simulink model "sm_motor_grader_Blade"  (R2025b)
settings: Solver=ode23t  StartTime=0.0  StopTime=stopTime  RelTol=1e-3  AbsTol=1e-3  EnableMultiTasking=on
undefined symbols (not defined in the file): activeTestCmds, motGradParams, X, Y, Z
libraries: sm_motor_grader_lib x4, sm_lib x4, nesl_utility x1, simulink x1
Description:
  | Copyright 2025 The MathWorks, Inc.
settings Model: Creator=smiller  LastModifiedBy=smiller
settings SolverCC: AutoScaleAbsTol=off  AlgebraicLoopSolver=TrustRegion  MaxZcPerStep=1.0
settings DataIOCC: LimitDataPoints=on  MaxDataPoints=10000  ReturnWorkspaceOutputs=off  SignalLoggingName=logsout_sm_motor_grader_Blade
settings OptimizationCC: ReuseModelBlockBuffer=off  LifeSpan=inf
settings DebuggingCC: UnconnectedInputMsg=warning  UnconnectedOutputMsg=warning  UnconnectedLineMsg=warning  AllowSymbolicDim=off  SubsystemReferenceDiagnosticForUnitTest=warning  SFUnexpectedBacktrackingDiag=warning  SFNoUnconditionalDefaultTransitionDiag=warning  SFExecutionAtInitializationDiag=none  ArithmeticOperatorsInVariantConditions=warning
settings ModelReferenceCC: EnableRefExpFcnMdlSchedulingChecks=on
settings SFSimCC: SimUseLocalCustomCode=off  CustomCodeUndefinedFunction=UseInterfaceOnly
settings RTWCC: RTWUseLocalCustomCode=off  GPUComputeCapability=3.5  DLArmComputeVersion=19.05
settings CodeAppCC: StateflowObjectComments=on
settings GRTTargetCC: TargetLangStandard=C89/C90 (ANSI)
settings ConfigComp: CovMetricSettings=dw  CovSaveCumulativeToWorkspaceVar=on  CovSaveSingleToWorkspaceVar=on  CovExternalEMLEnable=off  CovSFcnEnable=off
settings SimscapeCC: SimscapeLogType=all  SimscapeLogSimulationStatistics=on  SimscapeLogName=simlog_sm_motor_grader_Blade  SimscapeLogLimitData=off  SimscapeLogDataHistory=10000.0
settings DiagnosticsConfigSet: SimMechanicsConflictingReferenceFrames=none
settings ExplorerConfigSet: InternalSimMechanicsExplorerSettings="<ExplorerConfiguration><canonicalview>default</canonicalview><AnimationSetting><BasePlaybackSpeed>1.0</BasePlaybackSpeed><PlaybackSpeedFactor>1.0</PlaybackSpeedFactor></AnimationSetting><TilePanel><TileInfo><Tiles Columns=\"1\" Count=\"1\" Rows=\"1\"><Column Weight=\"1\"/><Row Weight=\"1\"/><Tile Height=\"1\" Width=\"1\" X=\"0\" Y=\"0\"/></Tiles></TileInfo><SceneInfo><SceneViewer><BGColor><R>1</R><G>1</G><B>1</B></BGColor><Camera><DoPerspective>off</DoPerspective><Position><X>-3.46230362549575776</X><Y>-2.62208562860429995</Y><Z>1.68751467196826876</Z></Position><Center><X>-0.265224461381971088</X><Y>0.208729678692644943</Y><Z>0.662364084836305378</Z></Center><Up><X>0.210150762827159998</X><Y>0.114284437926875038</Y><Z>0.970966386715266694</Z></Up><ViewLimDist>1</ViewLimDist><YLim>1.31618735358919769</YLim><XLim>2.34560763013940843</XLim></Camera></SceneViewer></SceneInfo></TilePanel><MechEditorPanel><Cameras/><GfxPanelCameraMap/><VideoCreator><PlaybackSpeedRatio>1.0</PlaybackSpeedRatio><FrameRate>30</FrameRate><VideoFormat>MPEG-4</VideoFormat><FrameSize>auto</FrameSize></VideoCreator></MechEditorPanel></ExplorerConfiguration>"

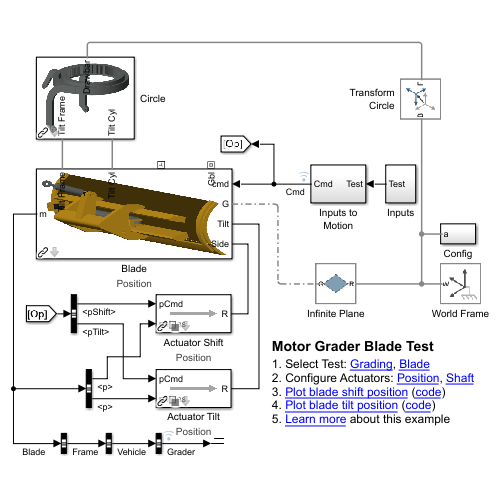
[thumbnail: Simulink's stored preview of the top-level diagram]
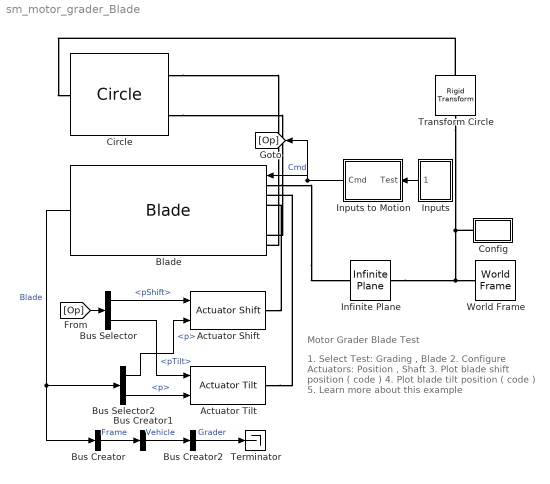
== system sm_motor_grader_Blade ==
  note: 1. Select Test: Grading , Blade
      | 2. Configure Actuators: Position , Shaft
      | 3. Plot blade shift position ( code )
      | 4. Plot blade tilt position ( code )
      | 5. Learn more about this example
  note: Motor Grader Blade Test
  Actuator Shift : sm_motor_grader_lib/Actuation/Actuator Shift  VariantControl=Actuator Shift  LabelModeActiveChoice=Position
      settings: AttributesFormatString=%<LabelModeActiveChoice>
  Actuator Tilt : sm_motor_grader_lib/Actuation/Actuator Tilt  VariantControl=Actuator Tilt  LabelModeActiveChoice=Position
      settings: AttributesFormatString=%<LabelModeActiveChoice>
  Blade : sm_motor_grader_lib/Blade  popup_actuator_model=Position  popup_blade_ground_contact=None
      settings: AttributesFormatString=%<popup_actuator_model>
  Bus Creator : BusCreator  Inputs=1
  Bus Creator1 : BusCreator  Inputs=1
  Bus Creator2 : BusCreator  Inputs=1
  Bus Selector : BusSelector  OutputSignals=pShift,pTilt
  Bus Selector2 : BusSelector  OutputSignals=Shift.p,Tilt.p
  Circle : sm_motor_grader_lib/Circle
  Config : Subsystem
  Infinite Plane : sm_lib/Curves and Surfaces/Infinite Plane  GraphicType=Rectangle  GraphicPlaneWidth=2  GraphicPlaneWidthUnits=m  GraphicPlaneHeight=8  GraphicPlaneHeightUnits=m  GraphicVisPropType=SimpleVisualProperties  GraphicDiffuseColor=[0.8 0.8 0.8]  GraphicOpacity=0.7  GraphicSpecularColor=[0.5 0.5 0.5 1.0]  GraphicAmbientColor=[0.15 0.15 0.15 1.0]  GraphicEmissiveColor=[0.0 0.0 0.0 1.0]  GraphicShininess=75
  Inputs : Subsystem
  Inputs to Motion : Subsystem
  Terminator : Terminator
  Transform Circle : sm_lib/Frames and Transforms/Rigid Transform  RotationMethod=StandardAxis  FollAlignAxisA=+X  BaseAlignAxisA=+Y  FollAlignAxisB=+Y  BaseAlignAxisB=+Z  RotationStandardAxis=+Z  RotationAngle=-90  RotationAngleUnits=deg  RotationArbitraryAxis=[0 0 1]  RotationSequenceAxes=FollowerAxes  RotationSequence=XYX  RotationSequenceAngles=[0 0 0]  RotationSequenceAnglesUnits=deg  RotationMatrix=[1 0 0;0 1 0;0 0 1]  Quaternion=[1 0 0 0]  TranslationMethod=StandardAxis  TranslationCartesianOffset=[0 0 0]  TranslationCartesianOffsetUnits=m  TranslationStandardAxis=+Z  TranslationStandardOffset=1.2109  TranslationStandardOffsetUnits=m  TranslationROffset=0  TranslationROffsetUnits=m  TranslationThetaOffset=0  TranslationThetaOffsetUnits=deg  TranslationZOffset=0  TranslationZOffsetUnits=m
  World Frame : sm_lib/Frames and Transforms/World Frame
  wires:
  Blade/1 -> Bus Creator/1, Bus Selector2/1  "Blade"
  Bus Creator/1 -> Bus Creator1/1  "Frame"
  Bus Creator1/1 -> Bus Creator2/1  "Vehicle"
  Inputs to Motion/1(Cmd) -> Blade/1, [Op]  "Cmd"
  [Op] -> Bus Selector/1
  Bus Selector/2 -> Actuator Tilt/1  "<pTilt>"
  Bus Selector2/2 -> Actuator Tilt/2  "<p>"
  Bus Selector2/1 -> Actuator Shift/2  "<p>"
  Bus Selector/1 -> Actuator Shift/1  "<pShift>"
  Inputs/1(Test) -> Inputs to Motion/1(Test)
  Bus Creator2/1 -> Terminator/1  "Grader"
  connections:
  Circle/RConn1 -- Blade/LConn7
  Circle/RConn2 -- Blade/LConn6
  Blade/LConn1 -- Infinite Plane/RConn1
  Actuator Tilt/RConn1 -- Blade/LConn2
  Actuator Shift/RConn1 -- Blade/LConn3
  Transform Circle/RConn1 -- Circle/LConn1
  Transform Circle/LConn1 -- Infinite Plane/LConn1 -- World Frame/RConn1 -- Config/RConn1

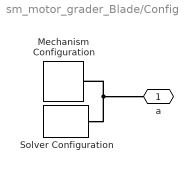
== system sm_motor_grader_Blade/Config ==
  Mechanism Configuration : sm_lib/Utilities/Mechanism Configuration  UniformGravity=Constant  GravityVector=[0 0 -9.80665]  GravityVectorUnits=m/s^2  LinearizationDelta=0.001  JointModeTransitionNonlinearIterations=2
  Solver Configuration : nesl_utility/Solver Configuration  PhysicalDomain=network_engine_domain  SubClassName=solver  LeftPortType=input  RightPortType=generic  Tones=[]  Harmonics=[]  SimulateNoise=off  Profile=off  UseLocalSampling=off  EnableSwitchedLinearOptims=on  FrequencyDomain=off  UseCCode=off  RelTol=0.001  AbsTol=0.001  MinStep=1e-09  ToWorkspace=off  RevertToSquareIcSolve=off  NumHomotopyIterations=100  PhasorMode=off  PhasorModeNumHarmonics=1  ConsistencySolver=NEWTON_XTOL_AFTER_FTOL  IndexReductionMethod=DerivativeReplacement  DoDC=off  ResidualTolerance=1e-09  ConsistencyTolSource=GLOBAL  ConsistencyAbsTol=0.001  ConsistencyRelTol=0.001  ConsistencyTolFactor=0.001  UseLocalSolver=off  LocalSolverChoice=NE_BACKWARD_EULER_ADVANCER  ResolveIndetEquations=on  FunctionEvalNumThread=1  LocalSolverSampleTime=0.001  DoFixedCost=off  MaxNonlinIter=3  MaxModeIter=2  ComputeImpulses=off  ImpulseIterations=2  LinearAlgebra=auto  LinearAlgebraNumThread=0  EquationFormulation=NE_TIME_EF  DelaysMemoryBudget=1024  AutomaticFiltering=on  FilteringTimeConstant=0.001  PartitionStorageMethod=AS_NEEDED  PartitionMemoryBudget=1024  PartitionMethod=ROBUST  MultibodyUseLocalSolver=off  MultibodyLocalSolverChoice=ODE1  MultibodyLocalSolverSampleTime=0.001
  a : PMIOPort  Side=Right
  connections:
  Solver Configuration/RConn1 -- a/RConn1 -- Mechanism Configuration/RConn1

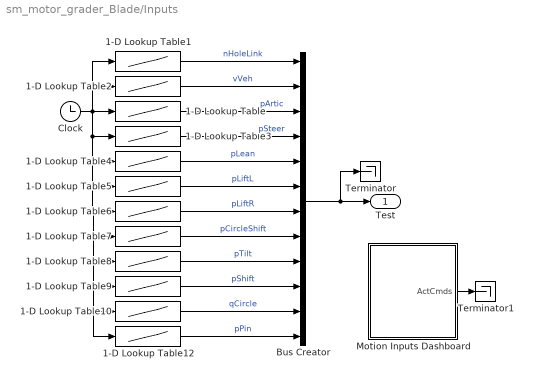
== system sm_motor_grader_Blade/Inputs ==
  1-D Lookup Table : Lookup_n-D  NumberOfTableDimensions=1  BreakpointsForDimension1=activeTestCmds.get('pArtic').Time  Table=activeTestCmds.get('pArtic').Data  InternalRulePriority=Speed  RndMeth=Simplest
  1-D Lookup Table1 : Lookup_n-D  NumberOfTableDimensions=1  BreakpointsForDimension1=activeTestCmds.get('nHoleLink').Time  Table=activeTestCmds.get('nHoleLink').Data  InternalRulePriority=Speed  RndMeth=Simplest
  1-D Lookup Table10 : Lookup_n-D  NumberOfTableDimensions=1  BreakpointsForDimension1=activeTestCmds.get('qCircle').Time  Table=activeTestCmds.get('qCircle').Data  InternalRulePriority=Speed  RndMeth=Simplest
  1-D Lookup Table12 : Lookup_n-D  NumberOfTableDimensions=1  BreakpointsForDimension1=activeTestCmds.get('pPin').Time  Table=activeTestCmds.get('pPin').Data  InternalRulePriority=Speed  RndMeth=Simplest
  1-D Lookup Table2 : Lookup_n-D  NumberOfTableDimensions=1  BreakpointsForDimension1=activeTestCmds.get('vVeh').Time  Table=activeTestCmds.get('vVeh').Data  InternalRulePriority=Speed  RndMeth=Simplest
  1-D Lookup Table3 : Lookup_n-D  NumberOfTableDimensions=1  BreakpointsForDimension1=activeTestCmds.get('pSteer').Time  Table=activeTestCmds.get('pSteer').Data  InternalRulePriority=Speed  RndMeth=Simplest
  1-D Lookup Table4 : Lookup_n-D  NumberOfTableDimensions=1  BreakpointsForDimension1=activeTestCmds.get('pLean').Time  Table=activeTestCmds.get('pLean').Data  InternalRulePriority=Speed  RndMeth=Simplest
  1-D Lookup Table5 : Lookup_n-D  NumberOfTableDimensions=1  BreakpointsForDimension1=activeTestCmds.get('pLiftL').Time  Table=activeTestCmds.get('pLiftL').Data  InternalRulePriority=Speed  RndMeth=Simplest
  1-D Lookup Table6 : Lookup_n-D  NumberOfTableDimensions=1  BreakpointsForDimension1=activeTestCmds.get('pLiftR').Time  Table=activeTestCmds.get('pLiftR').Data  InternalRulePriority=Speed  RndMeth=Simplest
  1-D Lookup Table7 : Lookup_n-D  NumberOfTableDimensions=1  BreakpointsForDimension1=activeTestCmds.get('pCircleShift').Time  Table=activeTestCmds.get('pCircleShift').Data  InternalRulePriority=Speed  RndMeth=Simplest
  1-D Lookup Table8 : Lookup_n-D  NumberOfTableDimensions=1  BreakpointsForDimension1=activeTestCmds.get('pTilt').Time  Table=activeTestCmds.get('pTilt').Data  InternalRulePriority=Speed  RndMeth=Simplest
  1-D Lookup Table9 : Lookup_n-D  NumberOfTableDimensions=1  BreakpointsForDimension1=activeTestCmds.get('pShift').Time  Table=activeTestCmds.get('pShift').Data  InternalRulePriority=Speed  RndMeth=Simplest
  Bus Creator : BusCreator  Inputs=12
  Clock : Clock
  Motion Inputs Dashboard : Subsystem
  Terminator : Terminator
  Terminator1 : Terminator
  Test : Outport
  wires:
  Clock/1 -> 1-D Lookup Table1/1, 1-D Lookup Table2/1, 1-D Lookup Table/1, 1-D Lookup Table9/1, 1-D Lookup Table12/1, 1-D Lookup Table10/1, 1-D Lookup Table8/1, 1-D Lookup Table7/1, 1-D Lookup Table6/1, 1-D Lookup Table5/1, 1-D Lookup Table4/1, 1-D Lookup Table3/1
  1-D Lookup Table7/1 -> Bus Creator/8  "pCircleShift"
  1-D Lookup Table10/1 -> Bus Creator/11  "qCircle"
  1-D Lookup Table12/1 -> Bus Creator/12  "pPin"
  1-D Lookup Table1/1 -> Bus Creator/1  "nHoleLink"
  1-D Lookup Table4/1 -> Bus Creator/5  "pLean"
  1-D Lookup Table/1 -> Bus Creator/3  "pArtic"
  1-D Lookup Table5/1 -> Bus Creator/6  "pLiftL"
  1-D Lookup Table8/1 -> Bus Creator/9  "pTilt"
  1-D Lookup Table9/1 -> Bus Creator/10  "pShift"
  1-D Lookup Table3/1 -> Bus Creator/4  "pSteer"
  1-D Lookup Table6/1 -> Bus Creator/7  "pLiftR"
  1-D Lookup Table2/1 -> Bus Creator/2  "vVeh"
  Bus Creator/1 -> Test/1, Terminator/1
  Motion Inputs Dashboard/1(ActCmds) -> Terminator1/1

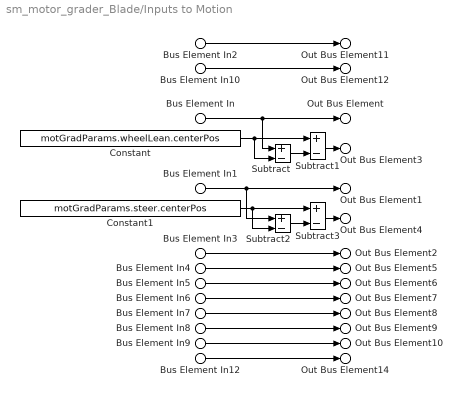
== system sm_motor_grader_Blade/Inputs to Motion ==
  Bus Element In : Inport  PortName=Test  Element=pLean
  Bus Element In1 : Inport  PortName=Test  Element=pSteer
  Bus Element In2 : Inport  PortName=Test  Element=vVeh
  Bus Element In3 : Inport  PortName=Test  Element=pArtic
  Bus Element In4 : Inport  PortName=Test  Element=pLiftL
  Bus Element In5 : Inport  PortName=Test  Element=pLiftR
  Bus Element In6 : Inport  PortName=Test  Element=pCircleShift
  Bus Element In7 : Inport  PortName=Test  Element=qCircle
  Bus Element In8 : Inport  PortName=Test  Element=pTilt
  Bus Element In9 : Inport  PortName=Test  Element=pShift
  Bus Element In10 : Inport  PortName=Test  Element=nHoleLink
  Bus Element In12 : Inport  PortName=Test  Element=pPin
  Constant : Constant  Value=motGradParams.wheelLean.centerPos
  Constant1 : Constant  Value=motGradParams.steer.centerPos
  Subtract{,1..3} (4 alike) : Sum  Inputs=+-
  Out Bus Element : Outport  PortName=Cmd  Element=pLeanL
  Out Bus Element1 : Outport  PortName=Cmd  Element=pSteerL
  Out Bus Element2 : Outport  PortName=Cmd  Element=pArtic
  Out Bus Element3 : Outport  PortName=Cmd  Element=pLeanR
  Out Bus Element4 : Outport  PortName=Cmd  Element=pSteerR
  Out Bus Element5 : Outport  PortName=Cmd  Element=pLiftL
  Out Bus Element6 : Outport  PortName=Cmd  Element=pLiftR
  Out Bus Element7 : Outport  PortName=Cmd  Element=pCircleShift
  Out Bus Element8 : Outport  PortName=Cmd  Element=qCircle
  Out Bus Element9 : Outport  PortName=Cmd  Element=pTilt
  Out Bus Element10 : Outport  PortName=Cmd  Element=pShift
  Out Bus Element11 : Outport  PortName=Cmd  Element=vVeh
  Out Bus Element12 : Outport  PortName=Cmd  Element=nHoleLink
  Out Bus Element14 : Outport  PortName=Cmd  Element=pPin
  wires:
  Bus Element In/1 -> Subtract/1, Out Bus Element/1
  Subtract1/1 -> Out Bus Element3/1
  Subtract3/1 -> Out Bus Element4/1
  Subtract/1 -> Subtract1/2
  Bus Element In1/1 -> Subtract2/1, Out Bus Element1/1
  Constant/1 -> Subtract/2, Subtract1/1
  Subtract2/1 -> Subtract3/2
  Constant1/1 -> Subtract2/2, Subtract3/1
  Bus Element In2/1 -> Out Bus Element11/1
  Bus Element In3/1 -> Out Bus Element2/1
  Bus Element In4/1 -> Out Bus Element5/1
  Bus Element In5/1 -> Out Bus Element6/1
  Bus Element In6/1 -> Out Bus Element7/1
  Bus Element In7/1 -> Out Bus Element8/1
  Bus Element In8/1 -> Out Bus Element9/1
  Bus Element In9/1 -> Out Bus Element10/1
  Bus Element In10/1 -> Out Bus Element12/1
  Bus Element In12/1 -> Out Bus Element14/1

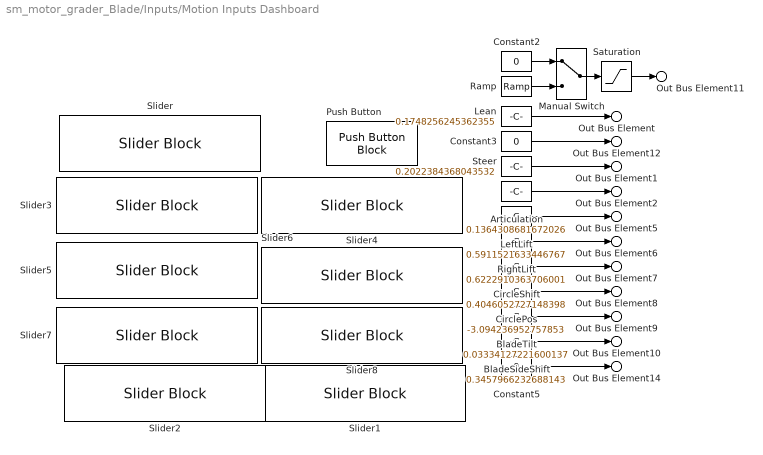
== system sm_motor_grader_Blade/Inputs/Motion Inputs Dashboard ==
  Articulation : Constant  Value=0.1364308681672026
  BladeSideShift : Constant  Value=0.3457966232688143
  BladeTilt : Constant  Value=0.03334127221600137
  CirclePos : Constant  Value=-3.094236952757853
  CircleShift : Constant  Value=0.4046052727148398
  Constant2 : Constant  Value=0
  Constant3 : Constant  Value=0
  Constant5 : Constant  Value=0
  Lean : Constant  Value=0.1748256245362355
  LeftLift : Constant  Value=0.5911521633446767
  Manual Switch : ManualSwitch
  Push Button : PushButtonBlock  ButtonText=Articulation  OnValue=0.126511  ButtonType=Latch  IconOnColor=[0.0, 0.39215686274509803, 0.0]  IconOffColor=[0.0, 1.0, 0.0]  OffValue=0.117183
  Ramp : simulink/Sources/Ramp  slope=0.5  start=5  InitialOutput=0
  RightLift : Constant  Value=0.6222910363706001
  Saturation : Saturate  UpperLimit=motGradParams.drivetrain.topSpeed  LowerLimit=-motGradParams.drivetrain.topSpeed
  Slider : SliderBlock  ScaleMin=0.05  ScaleMax=0.19
  Slider1 : SliderBlock  ScaleMin=0.15  ScaleMax=0.25
  Slider2 : SliderBlock  ScaleMin=0.14  ScaleMax=0.19
  Slider3 : SliderBlock  ScaleMax=1.2
  Slider4 : SliderBlock  ScaleMax=1.2
  Slider5 : SliderBlock  ScaleMax=0.85
  Slider6 : SliderBlock  ScaleMin=-90  ScaleMax=90
  Slider7 : SliderBlock  ScaleMax=0.2
  Slider8 : SliderBlock  ScaleMax=1.1
  Steer : Constant  Value=0.2022384368043532
  Out Bus Element : Outport  PortName=ActCmds  Element=pLean
  Out Bus Element1 : Outport  PortName=ActCmds  Element=pSteer
  Out Bus Element2 : Outport  PortName=ActCmds  Element=pArtic
  Out Bus Element5 : Outport  PortName=ActCmds  Element=pLiftL
  Out Bus Element6 : Outport  PortName=ActCmds  Element=pLiftR
  Out Bus Element7 : Outport  PortName=ActCmds  Element=pCircleShift
  Out Bus Element8 : Outport  PortName=ActCmds  Element=qCircle
  Out Bus Element9 : Outport  PortName=ActCmds  Element=pTilt
  Out Bus Element10 : Outport  PortName=ActCmds  Element=pShift
  Out Bus Element11 : Outport  PortName=ActCmds  Element=vVeh
  Out Bus Element12 : Outport  PortName=ActCmds  Element=nHoleLink
  Out Bus Element14 : Outport  PortName=ActCmds  Element=pPin
  wires:
  Ramp/1 -> Manual Switch/2
  Saturation/1 -> Out Bus Element11/1
  Constant2/1 -> Manual Switch/1
  Manual Switch/1 -> Saturation/1
  LeftLift/1 -> Out Bus Element5/1
  RightLift/1 -> Out Bus Element6/1
  CircleShift/1 -> Out Bus Element7/1
  CirclePos/1 -> Out Bus Element8/1
  BladeTilt/1 -> Out Bus Element9/1
  BladeSideShift/1 -> Out Bus Element10/1
  Lean/1 -> Out Bus Element/1
  Steer/1 -> Out Bus Element1/1
  Articulation/1 -> Out Bus Element2/1
  Constant3/1 -> Out Bus Element12/1
  Constant5/1 -> Out Bus Element14/1
